simulink model "lab2_1"  (R2020b)
settings: Solver=ode45  StartTime=0.0  StopTime=50  RelTol=1e-13
values from neighbouring files (symbols this model uses):
  g_l = g/l    (= 4.905)    [lab2.m]
  theta0 = 0 + 5*pi/180    (= 0.0872664625997)    [lab2.m]
  theta_dot0 = 0    [lab2.m]
settings Model: Creator=whitehole  LastModifiedBy=whitehole

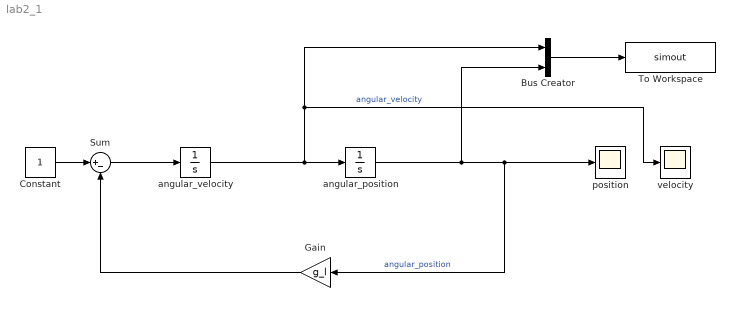
== system lab2_1 ==
  Bus Creator : BusCreator  Inputs=2
  Constant : Constant
  Gain : Gain  Gain=g_l
  Sum : Sum  Inputs=|+-
  To Workspace : ToWorkspace  VariableName=simout  SaveFormat=Timeseries  SampleTime=-1
  angular_position : Integrator  InitialCondition=theta0
  angular_velocity : Integrator  InitialCondition=theta_dot0
  position : Scope
  velocity : Scope
  wires:
  Constant/1 -> Sum/1
  angular_velocity/1 -> angular_position/1, Bus Creator/1, velocity/1  "angular_velocity"
  Sum/1 -> angular_velocity/1
  angular_position/1 -> Bus Creator/2, position/1, Gain/1  "angular_position"
  Gain/1 -> Sum/2
  Bus Creator/1 -> To Workspace/1
